simulink model "Lab2_1"  (R2016b)
settings: Solver=ode45  StartTime=0.0  StopTime=10.0  RelTol=1e-3
model workspace: external: MAT-File C:\Users\ag883_000\Documents\MATLAB\Lab2_3.mat (data not in the file)
values from neighbouring files (symbols this model uses):
  Bm = 500*10^-6    (= 0.0005)    [Lab2_2.m]
  iaic = simout(:,2)    [Lab2_2.m]
  Jtot = Jmotor + Jload    (= 0.7)    [Lab2_2.m]
  KL = 12*10^-6    (= 1.2e-05)    [Lab2_2.m]
  Kv = .0631    (= 0.0631)    [Lab2_2.m]
  La = .000014    (= 1.4e-05)    [Lab2_2.m]
  Ra = .0325    (= 0.0325)    [Lab2_2.m]
  va = 24    [Lab2_2.m]
  wmic = simout(:,3)    [Lab2_2.m]
settings Model: Creator=Andrew  LastModifiedBy=ag883_000

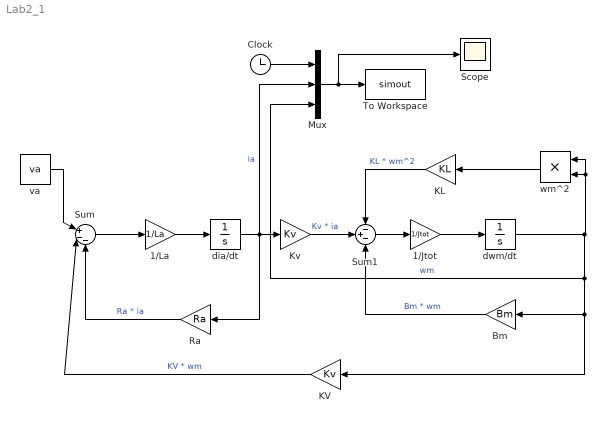
== system Lab2_1 ==
  1/Jtot : Gain  Gain=1/Jtot
  1/La : Gain  Gain=1/La
  Bm : Gain  Gain=Bm
  Clock : Clock
  KL : Gain  Gain=KL
  KV : Gain  Gain=Kv
  Kv : Gain  Gain=Kv
  Mux : Mux  Inputs=3
  Ra : Gain  Gain=Ra
  Scope : Scope
  Sum : Sum  Inputs=|+--
  Sum1 : Sum  Inputs=-+-
  To Workspace : ToWorkspace  VariableName=simout  SampleTime=-1
  dia/dt : Integrator  InitialCondition=iaic
  dwm/dt : Integrator  InitialCondition=wmic
  va : Constant  Value=va
  wm^2 : Product
  wires:
  Sum/1 -> 1/La/1
  1/La/1 -> dia/dt/1
  dia/dt/1 -> Mux/2, Ra/1, Kv/1  "ia"
  1/Jtot/1 -> dwm/dt/1
  dwm/dt/1 -> Mux/3, KV/1, Bm/1, wm^2/2, wm^2/1  "wm"
  wm^2/1 -> KL/1
  KV/1 -> Sum/2  "KV * wm"
  Ra/1 -> Sum/3  "Ra * ia"
  Kv/1 -> Sum1/2  "Kv * ia"
  KL/1 -> Sum1/1  "KL * wm^2"
  Sum1/1 -> 1/Jtot/1
  Bm/1 -> Sum1/3  "Bm * wm"
  va/1 -> Sum/1
  Mux/1 -> Scope/1, To Workspace/1
  Clock/1 -> Mux/1
